simulink subsystem "simplified_datetime_modelling_and_ref_frames"  (R2024a)
settings: Solver=VariableStepAuto  StartTime=0.0  StopTime=10.0  RelTol=1e-3
undefined symbols (not defined in the file or in its folder): IAU
libraries: simulink_extras x1, aerolibtransform2 x1, aerolibutil x1
settings Model: Creator=joshu  LastModifiedBy=joshu

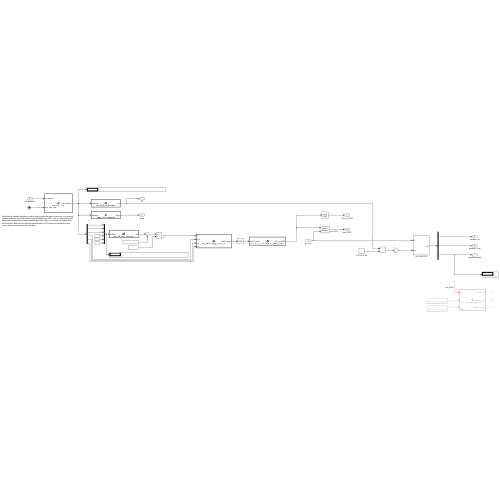
[thumbnail: Simulink's stored preview of the top-level diagram]
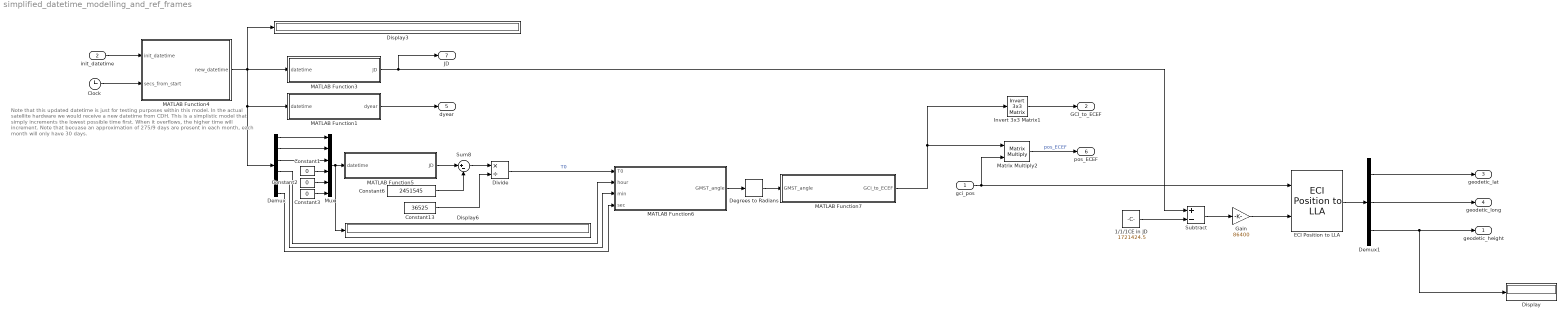
== system simplified_datetime_modelling_and_ref_frames ==
  note: Note that this updated datetime is just for testing purposes within this model. In the actual satellite hardware we would receive a new datetime from CDH. This is a simplistic model that simply increments the lowest possible time first. When it overflows, the higher time will increment. Note that becuase an approximation of 275/9 days are present in each month, each month will only have 30 days.
  gci_pos : Inport
  init_datetime : Inport  Port=2
  1/1/1CE in JD : Constant  Value=1721424.5
  Clock : Clock
  Constant1 : Constant  Value=0
  Constant13 : Constant  Value=36525
  Constant2 : Constant  Value=0
  Constant3 : Constant  Value=0
  Constant6 : Constant  Value=2451545
  Degrees to Radians : simulink_extras/Transformations/Degrees to Radians
  Demux : Demux  Outputs=6
  Demux1 : Demux  Outputs=3
  Display : Display
  Display3 : Display
  Display6 : Display
  Divide : Product  Inputs=*/
  ECI Position to LLA : aerolibtransform2/ECI Position to LLA  red=IAU-2000/2006  year=1  month=January  day=1  hour=0  min=0  sec=0  deltaT=Sec  errorflag=None  extraparamflag=off  eunits=Metric (MKS)  earthmodel=WGS84  flat=1/298.257223563  eqradius=6378137
      settings: AttributesFormatString=%<red>
  Gain : Gain  Gain=86400
  Invert 3x3 Matrix1 : aerolibutil/Invert  3x3 Matrix
  MATLAB Function1 : MATLAB Function  TreatAsAtomicUnit=on
  MATLAB Function3 : MATLAB Function  TreatAsAtomicUnit=on
  MATLAB Function4 : MATLAB Function  TreatAsAtomicUnit=on
  MATLAB Function5 : MATLAB Function  TreatAsAtomicUnit=on
  MATLAB Function6 : MATLAB Function  TreatAsAtomicUnit=on
  MATLAB Function7 : MATLAB Function  TreatAsAtomicUnit=on
  Matrix Multiply2 : Product  Multiplication=Matrix(*)
  Mux : Mux  Inputs=6
  Subtract : Sum  Inputs=+-
  Sum8 : Sum  Inputs=|+-
  geodetic_height : Outport
  GCI_to_ECEF : Outport  Port=2
  geodetic_lat : Outport  Port=3
  geodetic_long : Outport  Port=4
  dyear : Outport  Port=5
  pos_ECEF : Outport  Port=6
  JD : Outport  Port=7
  wires:
  Constant3/1 -> Mux/6
  Demux1/1 -> geodetic_lat/1
  Divide/1 -> MATLAB Function6/1(T0)  "T0"
  MATLAB Function4/1(new_datetime) -> Display3/1, MATLAB Function3/1(datetime), Demux/1, MATLAB Function1/1(datetime)
  MATLAB Function6/1(GMST_angle) -> Degrees to Radians/1
  MATLAB Function1/1(dyear) -> dyear/1
  Invert 3x3 Matrix1/1 -> GCI_to_ECEF/1
  MATLAB Function3/1(JD) -> JD/1, Subtract/1
  Demux1/3 -> geodetic_height/1, Display/1
  Demux1/2 -> geodetic_long/1
  Constant1/1 -> Mux/4
  Demux/5 -> MATLAB Function6/3(min)
  Demux/1 -> Mux/1
  Sum8/1 -> Divide/1
  Constant13/1 -> Divide/2
  Matrix Multiply2/1 -> pos_ECEF/1  "pos_ECEF"
  Demux/6 -> MATLAB Function6/4(sec)
  Constant6/1 -> Sum8/2
  gci_pos/1 -> ECI Position to LLA/1, Matrix Multiply2/2
  MATLAB Function5/1(JD) -> Sum8/1
  MATLAB Function7/1(GCI_to_ECEF) -> Matrix Multiply2/1, Invert 3x3 Matrix1/1
  Degrees to Radians/1 -> MATLAB Function7/1(GMST_angle)
  Mux/1 -> MATLAB Function5/1(datetime), Display6/1
  init_datetime/1 -> MATLAB Function4/1(init_datetime)
  Clock/1 -> MATLAB Function4/2(secs_from_start)
  Demux/3 -> Mux/3
  Demux/4 -> MATLAB Function6/2(hour)
  Demux/2 -> Mux/2
  Constant2/1 -> Mux/5
  Subtract/1 -> Gain/1
  Gain/1 -> ECI Position to LLA/2
  1/1/1CE in JD/1 -> Subtract/2
  ECI Position to LLA/1 -> Demux1/1

== matlab function simplified_datetime_modelling_and_ref_frames/MATLAB Function1 ==
  data: datetime input; dyear output
function dyear = dyear_from_datetime(datetime)

    % the datetime format is provided as a 6 value array
    % year, month, day, hour, minute, second

    % sequentially builds the decimal year

    % potentially we may want to use /61 for leap second days but this is
    % likely fine as our simulation just needs to perform regular datetime
    % updates for simple testing

    tot_mins = datetime(5) + datetime(6) / 60;
    tot_hours = datetime(4) + tot_mins / 60;
    tot_days = datetime(3) + tot_hours / 24;
    tot_months = datetime(2) + tot_days / (275/9); % average days in month across year
    tot_years = datetime(1) + tot_months / 12;

    dyear = tot_years;

== matlab function simplified_datetime_modelling_and_ref_frames/MATLAB Function3 ==
  data: datetime input; JD output
function JD = calc_JD_from_datetime(datetime)

% the datetime format is provided as a 6 value array
% year, month, day, hour, minute, second

% calculates the Julian date (JD) from the datetime
JD = 1721013.5 + 367*datetime(1) - floor(7/4*(datetime(1) + ...
    floor((datetime(2) + 9)/12))) + floor(275/9*datetime(2)) + ...
    datetime(3) + (60*datetime(4) + datetime(5) + datetime(6)/60)/1440;

% note that seconds should be /61 for leap days but since we are using a
% testing environment we do not need to worry about this

% presumably in the navigation system of the actual satellite we may also
% not need to consider this as it would introduce a negligible error or we
% may need to have some special protocol with CDH to figure out a system

== matlab function simplified_datetime_modelling_and_ref_frames/MATLAB Function4 ==
  data: init_datetime input; new_datetime output; secs_from_start input
function new_datetime  = datetime_upd(init_datetime, secs_from_start)

% the datetime format is provided as a 6 value array
% year, month, day, hour, minute, second

% initializes new datetime array
new_datetime = zeros(1, 6);

% adds the seconds from start of simulation to seconds
new_datetime(6) = init_datetime(6) + secs_from_start;

% computes the new seconds and minutes with carry over
new_datetime(5) = init_datetime(5) + floor(new_datetime(6) / 60);
new_datetime(6) = mod(new_datetime(6), 60);

% computes the new minutes and hours with carry over
new_datetime(4) = init_datetime(4) + floor(new_datetime(5) / 60);
new_datetime(5) = mod(new_datetime(5), 60);

% computes the new hours and days with carry over
new_datetime(3) = init_datetime(3) + floor(new_datetime(4) / 24);
new_datetime(4) = mod(new_datetime(4), 24);

% computes the new days and months with carry over
new_datetime(2) = init_datetime(2) + floor(new_datetime(3) / (275/9));

% NOTE: the floor here is specifically needed to prevent a recurring
% decimal from occurring here due to using an average number of days per
% month of 275/9 (this also caps days in a month to 30)
new_datetime(3) = floor(mod(new_datetime(3), (275/9)));

% computes the new months and years with carry over

% for calculations, shifts first month to 0
new_datetime(2) = new_datetime(2) - 1;

new_datetime(1) = init_datetime(1) + floor(new_datetime(2) / 12);

% done with calculations, restores first month to 1
new_datetime(2) = mod(new_datetime(2), 12) + 1;

end

== matlab function simplified_datetime_modelling_and_ref_frames/MATLAB Function5 ==
  data: datetime input; JD output
function JD = calc_JD_from_datetime(datetime)

% the datetime format is provided as a 6 value array
% year, month, day, hour, minute, second

% calculates the Julian date (JD) from the datetime
JD = 1721013.5 + 367*datetime(1) - floor(7/4*(datetime(1) + ...
    floor((datetime(2) + 9)/12))) + floor(275/9*datetime(2)) + ...
    datetime(3) + (60*datetime(4) + datetime(5) + datetime(6)/60)/1440;

% note that seconds should be /61 for leap days but since we are using a
% testing environment we do not need to worry about this

% presumably in the navigation system of the actual satellite we may also
% not need to consider this as it would introduce a negligible error or we
% may need to have some special protocol with CDH to figure out a system

== matlab function simplified_datetime_modelling_and_ref_frames/MATLAB Function6 ==
  data: T0 input; GMST_angle output; hour input; min input; sec input
function GMST_angle = calc_GMST_angle_from_T0(T0, hour, min, sec)

% calculates GMST_angle in units of seconds (longitudinal seconds)
GMST_angle = 24110.54841 + 8640184.812866 * T0 + 0.093104 * T0^2 ...
    - 6.2e-6 * T0^3 + 1.002737909350795 * (3600*hour + 60*min + sec);

% reduces to range of 0-86400
GMST_angle = mod(GMST_angle, 86400);

% converts to degrees (there are 240 longitudinal seconds in a degree)
GMST_angle = GMST_angle / 240;

== matlab function simplified_datetime_modelling_and_ref_frames/MATLAB Function7 ==
  data: GMST_angle input; GCI_to_ECEF output
function GCI_to_ECEF = calc_GCI_to_ECEF_from_GMST_angle(GMST_angle)

% calculates the transformation matrix from GCI to ECEF
GCI_to_ECEF = [cos(GMST_angle) sin(GMST_angle) 0 ; ...
    -sin(GMST_angle) cos(GMST_angle) 0 ; 0 0 1];
